simulink model "OneParallel0NoActions"  (Simulink 9.0)
settings: Solver=ode45  StartTime=0.0  StopTime=10.0  RelTol=1e-3  EnableMultiTasking=on
settings Model: SuppressorTable=22 serialization::archive 11 0 6 0 0 0 0 0  Creator=scaife  LastModifiedBy=hbourbou  ExtModeAutoUpdateStatusClock=off
settings DataIOCC: LimitDataPoints=on  SignalLoggingSaveFormat=ModelDataLogs  SignalLoggingName=sigsOut
settings DebuggingCC: SaveWithParameterizedLinksMsg=none  SignalResolutionControl=TryResolveAllWithWarning  MultiTaskDSMMsg=warning  MultiTaskCondExecSysMsg=none
settings HardwareCC: TargetUnknown=on
settings SFSimCC: SimParseCustomCode=off
settings GRTTargetCC: CombineOutputUpdateFcns=off  GRTInterface=on

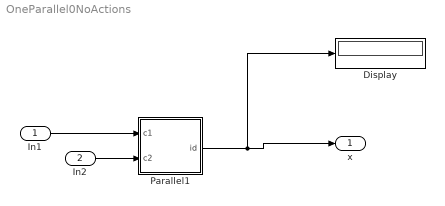
== system OneParallel0NoActions ==
  In1 : Inport  OutDataTypeStr=boolean
  In2 : Inport  Port=2  OutDataTypeStr=boolean
  Display : Display
  Parallel1 : Stateflow chart  TreatAsAtomicUnit=on
  x : Outport
  wires:
  Parallel1/1(id) -> Display/1, x/1
  In1/1 -> Parallel1/1(c1)
  In2/1 -> Parallel1/2(c2)

== stateflow chart Parallel1 ==
  state N1/ [parallel]
    en:id=1
    settings: executionOrder=1
    state B/
      en: id=22;
    state A/
      en: id=21;
    (default) -> A
    A -> B : [c1]
    B -> A : [c2]
  data: c1 input double; c2 input double; id output double
